simulink model "test"  (R2020a)
settings: Solver=FixedStepAuto  StartTime=0.0  StopTime=10  FixedStep=1e-3  RelTol=1e-3  EnableMultiTasking=on
libraries: frdmk64flib x1
settings Model: ExtModeTrigDuration=5  Creator=emily  LastModifiedBy=emily
settings OptimizationCC: EnhancedBackFolding=on  PassReuseOutputArgsAs=Individual arguments  ZeroExternalMemoryAtStartup=off  ZeroInternalMemoryAtStartup=off  MaxStackSize=64  OptimizeBlockOrder=speed  DifferentSizesBufferReuse=on  OptimizationCustomize=off  EfficientTunableParamExpr=on
settings DebuggingCC: ParameterTunabilityLossMsg=error
settings HardwareCC: ProdBitPerPointer=32  ProdBitPerSizeT=32  ProdBitPerPtrDiffT=32  ProdLargestAtomicInteger=Long  ProdLargestAtomicFloat=Double  ProdWordSize=32  ProdHWDeviceType=ARM Compatible->ARM Cortex
settings SFSimCC: MATLABDynamicMemAlloc=off
settings RTWCC: SystemTargetFile=ert.tlc  HardwareBoard=NXP FRDM-K64F  TemplateMakefile=ert_default_tmf  Toolchain=GNU Tools for ARM Embedded Processors
settings CodeAppCC: ForceParamTrailComments=on  IgnoreCustomStorageClasses=off  OperatorAnnotations=on  SimulinkDataObjDesc=on  SFDataObjDesc=on  InsertBlockDesc=on

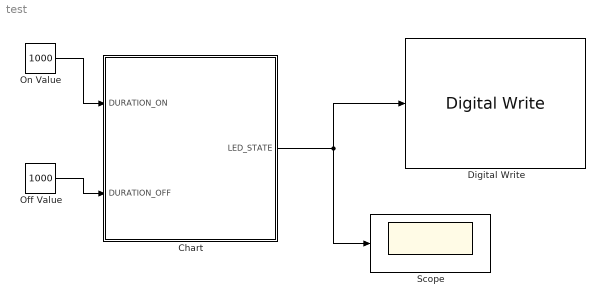
== system test ==
  Chart : Stateflow chart  TreatAsAtomicUnit=on
  Digital Write : frdmk64flib/Digital Write  Whichpin=RED_LED
  Off Value : Constant  Value=1000  OutDataTypeStr=int16
  On Value : Constant  Value=1000  OutDataTypeStr=int16
  Scope : Scope
  wires:
  Chart/1(LED_STATE) -> Digital Write/1, Scope/1
  On Value/1 -> Chart/1(DURATION_ON)
  Off Value/1 -> Chart/2(DURATION_OFF)

== stateflow chart test/Chart ==
  state LED_ON
    entry:
    LED_STATE=true;
  state LED_OFF
    entry:
    LED_STATE=false;
  (default) -> LED_ON
  LED_ON -> LED_OFF : after(DURATION_ON, msec)
  LED_OFF -> LED_ON : after(DURATION_OFF, msec)
  data: DURATION_ON input; DURATION_OFF input; LED_STATE output boolean
